simulink model "regelstrecke_simulink"  (R2025b)
settings: Solver=VariableStepAuto  StartTime=0.0  StopTime=10.0  MinStep=1e-3  RelTol=1e-3
values from neighbouring files (symbols this model uses):
  ci = 0.01    [params.m]
  cy = 1    [params.m]
  jump_end_val = 0    [p_regler.m]    (also in pd_regler.m; regelstrecke.m = 1)
  jump_init_val = 0    [p_regler.m]    (also in pd_regler.m; regelstrecke.m)
  jump_time = 0    [p_regler.m]    (also in pd_regler.m; regelstrecke.m)
  L = 0.1    [params.m]
  m = 10e-3    (= 0.01)    [params.m]
  R = 5    [params.m]
settings Model: Creator=rishabh  LastModifiedBy=rishabh

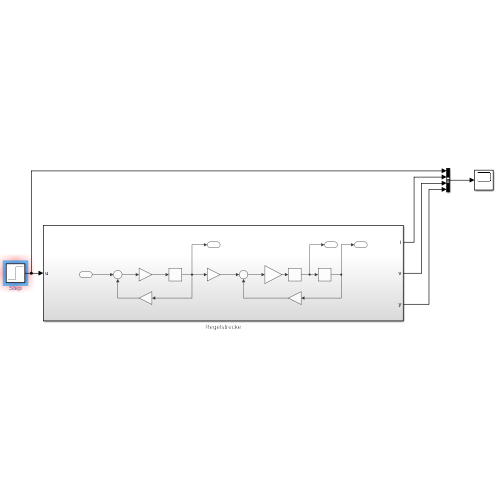
[thumbnail: Simulink's stored preview of the top-level diagram]
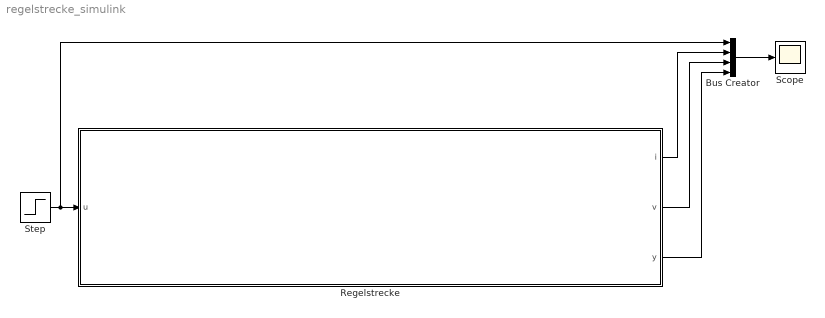
== system regelstrecke_simulink ==
  Bus Creator : BusCreator  Inputs=4
  Regelstrecke : Subsystem
  Scope : Scope
  Step : Step  Time=jump_time  Before=jump_init_val  After=jump_end_val  SampleTime=0
  wires:
  Step/1 -> Bus Creator/1, Regelstrecke/1(u)
  Bus Creator/1 -> Scope/1
  Regelstrecke/1(i) -> Bus Creator/2
  Regelstrecke/2(v) -> Bus Creator/3
  Regelstrecke/3(y) -> Bus Creator/4

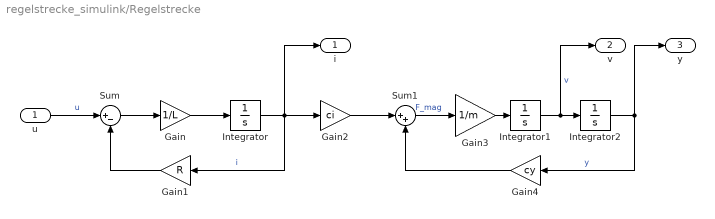
== system regelstrecke_simulink/Regelstrecke ==
  u : Inport
  Gain : Gain  Gain=1/L
  Gain1 : Gain  Gain=R
  Gain2 : Gain  Gain=ci
  Gain3 : Gain  Gain=1/m
  Gain4 : Gain  Gain=cy
  Integrator : Integrator
  Integrator1 : Integrator
  Integrator2 : Integrator
  Sum : Sum  Inputs=|+-
  Sum1 : Sum  Inputs=|++
  i : Outport
  v : Outport  Port=2
  y : Outport  Port=3
  wires:
  Gain1/1 -> Sum/2
  Sum/1 -> Gain/1
  Gain2/1 -> Sum1/1
  Gain/1 -> Integrator/1
  Gain3/1 -> Integrator1/1
  Integrator2/1 -> y/1, Gain4/1  "y"
  u/1 -> Sum/1  "u"
  Gain4/1 -> Sum1/2
  Integrator/1 -> i/1, Gain2/1, Gain1/1  "i"
  Sum1/1 -> Gain3/1  "F_mag"
  Integrator1/1 -> v/1, Integrator2/1  "v"
